simulink model "tetra_mod_qpsk"  (Simulink 8.0)
settings: Solver=FixedStepDiscrete  SolverMode=SingleTasking  StartTime=0.0  StopTime=1.0  RelTol=1e-3
undefined symbols (not defined in the file): figposition, Fs, get, sided, Two
libraries: commsink2 x4, simulink x2, commseqgen2 x2, commcnvcod2 x2, commdigbbndpm3 x2, commfilt2 x2, commrandsrc2 x1, commchan3 x1, dspsnks4 x1, dspvision x1
settings Model: Creator=tisc1101  LastModifiedBy=Dimav
settings DataIOCC: SignalLoggingSaveFormat=ModelDataLogs
settings DebuggingCC: FcnCallInpInsideContextMsg=UseLocalSettings
settings SFSimCC: SimParseCustomCode=off
settings GRTTargetCC: CombineOutputUpdateFcns=off  GRTInterface=on

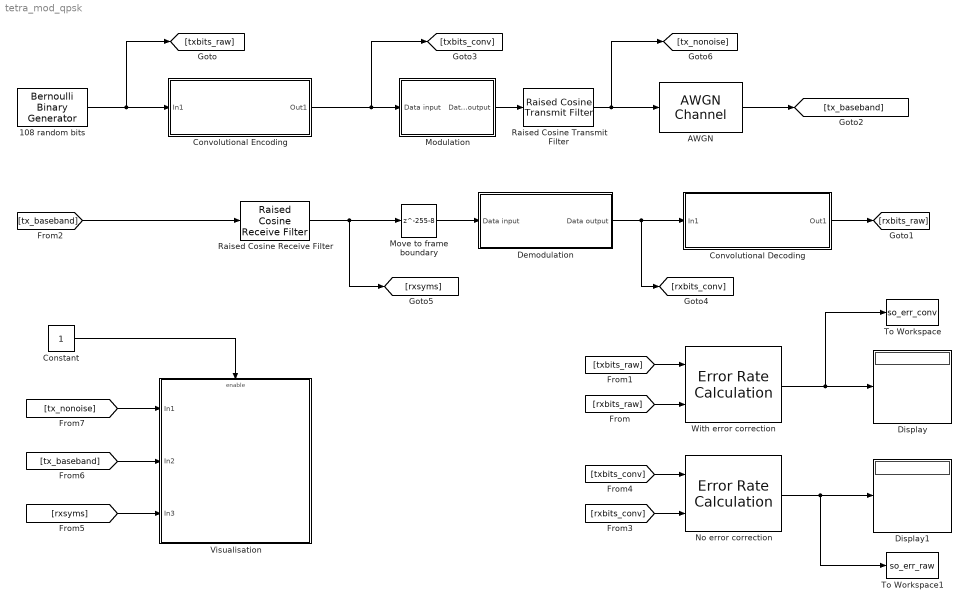
== system tetra_mod_qpsk ==
  108 random bits : commrandsrc2/Bernoulli Binary Generator  P=0.5  seed=61  Ts=1/(36000/512*108)  frameBased=on  sampPerFrame=108  orient=off  outDataType=double
  AWGN : commchan3/AWGN Channel  InputProcessing=Inherited (this choice will be removed - see release notes)  seed=67  noiseMode="Signal to noise ratio  (SNR)"  EbNodB=10  EsNodB=10  SNRdB=-10  bitsPerSym=1  Ps=1  Tsym=1  variance=1
  Constant : Constant
  Convolutional Decoding : Subsystem
  Convolutional Encoding : Subsystem
  Demodulation : Subsystem
  Display : Display
  Display1 : Display
  Modulation : Subsystem
  Move to frame boundary : Delay  DelayLength=255-8  InputProcessing=Inherited
  No error correction : commsink2/Error Rate Calculation  N=216  st_delay=0  cp_mode=Entire frame  subframe=[]  PMode=Port  WsName=ErrorVec  RsMode2=off  stop=off  numErr=100  maxBits=1e6
  Raised Cosine Receive Filter : commfilt2/Raised Cosine Receive Filter  filtType=Square root  N=8  D=4  R=0.35  sampMode=Mute  saveAsFlag=0  rateMode=Downsampling  downFactor=8  downOffset=0  framing=Maintain input frame rate  InputProcessing=Columns as channels (frame based)  checkGain=Normalized  filterGain=2  checkCoeff=off  variableName=rcRxFilt  launchFVT=off  roundingMode=Floor  overflowMode=off
  Raised Cosine Transmit Filter : commfilt2/Raised Cosine Transmit Filter  filtType=Square root  D=4  R=0.35  sampMode=Mute  saveAsFlag=0  N=8  framing=Maintain input frame rate  InputProcessing=Columns as channels (frame based)  checkGain=Normalized  filterGain=1  checkCoeff=off  variableName=rcTxFilt  launchFVT=off  roundingMode=Floor  overflowMode=off
  To Workspace : ToWorkspace  VariableName=so_err_conv  SampleTime=-1  SaveFormat=Structure
  To Workspace1 : ToWorkspace  VariableName=so_err_raw  SampleTime=-1  SaveFormat=Structure
  Visualisation : Subsystem  TreatAsAtomicUnit=on
  With error correction : commsink2/Error Rate Calculation  N=156  st_delay=0  cp_mode=Entire frame  subframe=[]  PMode=Port  WsName=ErrorVec  RsMode2=off  stop=off  numErr=100  maxBits=1e6
  wires:
  Modulation/1(Data output) -> Raised Cosine Transmit Filter/1
  Demodulation/1(Data output) -> [rxbits_conv], Convolutional Decoding/1(In1)
  [rxbits_raw] -> With error correction/2
  With error correction/1 -> Display/1, To Workspace/1
  Raised Cosine Transmit Filter/1 -> AWGN/1, [tx_nonoise]
  [tx_baseband] -> Raised Cosine Receive Filter/1
  Raised Cosine Receive Filter/1 -> Move to frame boundary/1, [rxsyms]
  Move to frame boundary/1 -> Demodulation/1(Data input)
  AWGN/1 -> [tx_baseband]
  Convolutional Encoding/1(Out1) -> Modulation/1(Data input), [txbits_conv]
  Convolutional Decoding/1(Out1) -> [rxbits_raw]
  [txbits_raw] -> With error correction/1
  [rxbits_conv] -> No error correction/2
  No error correction/1 -> Display1/1, To Workspace1/1
  [txbits_conv] -> No error correction/1
  108 random bits/1 -> Convolutional Encoding/1(In1), [txbits_raw]
  Constant/1 -> Visualisation/Enable
  [tx_baseband] -> Visualisation/2(In2)
  [rxsyms] -> Visualisation/3(In3)
  [tx_nonoise] -> Visualisation/1(In1)

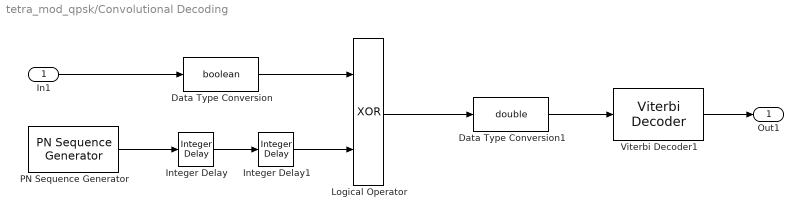
== system tetra_mod_qpsk/Convolutional Decoding ==
  In1 : Inport
  Data Type Conversion : DataTypeConversion  OutDataTypeStr=boolean
  Data Type Conversion1 : DataTypeConversion  OutDataTypeStr=double
  Integer Delay : simulink/Discrete/Integer Delay  NumDelays=215  InputProcessing=Inherited  vinit=0  samptime=-1
  Integer Delay1 : simulink/Discrete/Integer Delay  NumDelays=1  InputProcessing=Inherited  vinit=0  samptime=-1
  Logical Operator : Logic  Operator=XOR  AllPortsSameDT=off  OutDataTypeStr=boolean
  PN Sequence Generator : commseqgen2/PN Sequence Generator  poly=[1 1 1 0 1 1 0 1 1 0 1 1 1 0 0 0 1 0 0 0 0 0 1 1 0 0 1 0 0 0 0 0 1]  ini_sta=[0 1 0 1 0 1 0 1 0 1 0 1 0 1 0 1 0 1 0 1 0 1 0 1 0 1 0 1 0 1 1 1]  outBitMaskSource=Dialog parameter  shift=0  outVarSiz=off  maxOutSizeMode=Dialog parameter  maxOutSize=[10 1]  Ts=1/(36000/512*216)  frameBased=on  sampPerFrame=216  reset=off  bitPackedOutputs=off  outDataType=boolean  numPackedBits=8  bitPackDataSigned=off  bitPackedOutDType=double
  Viterbi Decoder1 : commcnvcod2/Viterbi Decoder  trellis=poly2trellis(7, [171 133])  isPunctured=off  punctureVector=[1; 1; 0; 1; 0; 1]  erasures=off  dectype=Hard decision  runSigValErrCheck=off  nsdecb=3  smWordLength=16  tbdepth=48  opmode=Continuous  reset=off  outDataType=double
  Out1 : Outport
  wires:
  Viterbi Decoder1/1 -> Out1/1
  Logical Operator/1 -> Data Type Conversion1/1
  In1/1 -> Data Type Conversion/1
  PN Sequence Generator/1 -> Integer Delay/1
  Data Type Conversion/1 -> Logical Operator/1
  Data Type Conversion1/1 -> Viterbi Decoder1/1
  Integer Delay/1 -> Integer Delay1/1
  Integer Delay1/1 -> Logical Operator/2

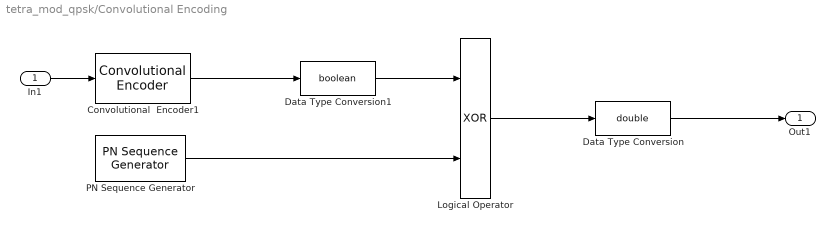
== system tetra_mod_qpsk/Convolutional Encoding ==
  In1 : Inport
  Convolutional  Encoder1 : commcnvcod2/Convolutional Encoder  trellis=poly2trellis(7, [171 133])  opMode=Continuous  DelayedResetAction=off  hasIniStPort=off  hasFinStPort=off  usePuncVector=off  punctureVector=[1; 1; 0; 1; 0; 1]  reset=Unused parameter value
  Data Type Conversion : DataTypeConversion  OutDataTypeStr=double
  Data Type Conversion1 : DataTypeConversion  OutDataTypeStr=boolean
  Logical Operator : Logic  Operator=XOR  AllPortsSameDT=off  OutDataTypeStr=boolean
  PN Sequence Generator : commseqgen2/PN Sequence Generator  poly=[1 1 1 0 1 1 0 1 1 0 1 1 1 0 0 0 1 0 0 0 0 0 1 1 0 0 1 0 0 0 0 0 1]  ini_sta=[0 1 0 1 0 1 0 1 0 1 0 1 0 1 0 1 0 1 0 1 0 1 0 1 0 1 0 1 0 1 1 1]  outBitMaskSource=Dialog parameter  shift=0  outVarSiz=off  maxOutSizeMode=Dialog parameter  maxOutSize=[10 1]  Ts=1/(36000/512*216)  frameBased=on  sampPerFrame=216  reset=off  bitPackedOutputs=off  outDataType=boolean  numPackedBits=8  bitPackDataSigned=off  bitPackedOutDType=double
  Out1 : Outport
  wires:
  In1/1 -> Convolutional  Encoder1/1
  Convolutional  Encoder1/1 -> Data Type Conversion1/1
  PN Sequence Generator/1 -> Logical Operator/2
  Logical Operator/1 -> Data Type Conversion/1
  Data Type Conversion/1 -> Out1/1
  Data Type Conversion1/1 -> Logical Operator/1

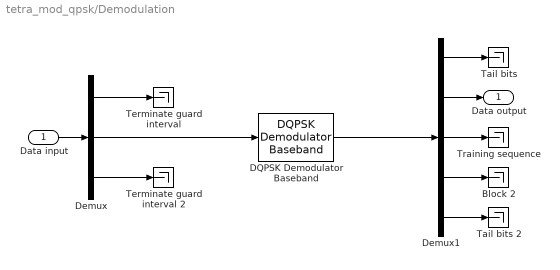
== system tetra_mod_qpsk/Demodulation ==
  Data input : Inport
  Block 2 : Terminator
  DQPSK Demodulator Baseband : commdigbbndpm3/DQPSK Demodulator Baseband  SystemSampleTime=-1  OutType=Bit  Dec=Gray  Ph=pi/4  outDtype1=Inherit via internal rule  outDtype2=Inherit via internal rule
  Demux : Demux  Outputs=[17 231 7]
  Demux1 : Demux  Outputs=[4 216 22 216 4]
  Tail bits : Terminator
  Tail bits 2 : Terminator
  Terminate guard interval : Terminator
  Terminate guard interval 2 : Terminator
  Training sequence : Terminator
  Data output : Outport
  wires:
  Demux/1 -> Terminate guard interval/1
  Demux/3 -> Terminate guard interval 2/1
  Demux/2 -> DQPSK Demodulator Baseband/1
  DQPSK Demodulator Baseband/1 -> Demux1/1
  Demux1/1 -> Tail bits/1
  Demux1/3 -> Training sequence/1
  Demux1/4 -> Block 2/1
  Demux1/5 -> Tail bits 2/1
  Data input/1 -> Demux/1
  Demux1/2 -> Data output/1

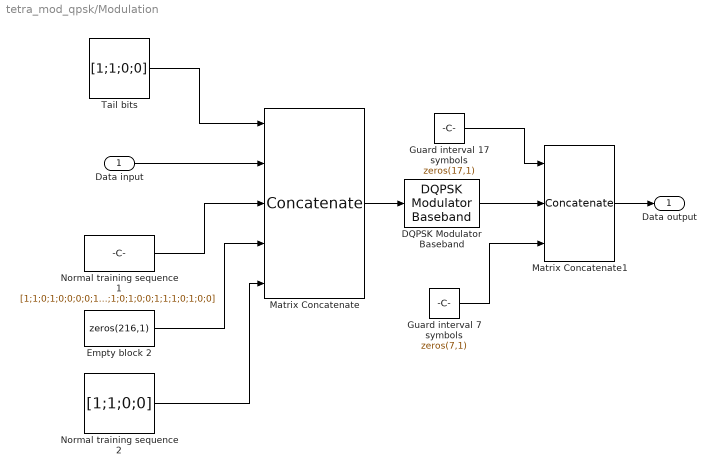
== system tetra_mod_qpsk/Modulation ==
  Data input : Inport
  DQPSK Modulator Baseband : commdigbbndpm3/DQPSK Modulator Baseband  SystemSampleTime=-1  InType=Bit  Enc=Gray  Ph=pi/4  outDtype=double
  Empty block 2 : Constant  Value=zeros(216,1)  VectorParams1D=off
      settings: SamplingMode=Frame based
  Guard interval 17 symbols : Constant  Value=zeros(17,1)  VectorParams1D=off
      settings: SamplingMode=Frame based
  Guard interval 7 symbols : Constant  Value=zeros(7,1)  VectorParams1D=off
      settings: SamplingMode=Frame based
  Matrix Concatenate : Concatenate  NumInputs=5  Mode=Multidimensional array
  Matrix Concatenate1 : Concatenate  NumInputs=3  Mode=Multidimensional array
  Normal training sequence 1 : Constant  Value=[1;1;0;1;0;0;0;0;1;1;1;0;1;0;0;1;1;1;0;1;0;0]  VectorParams1D=off
      settings: SamplingMode=Frame based
  Normal training sequence 2 : Constant  Value=[1;1;0;0]  VectorParams1D=off
      settings: SamplingMode=Frame based
  Tail bits : Constant  Value=[1;1;0;0]  VectorParams1D=off
      settings: SamplingMode=Frame based
  Data output : Outport
  wires:
  Tail bits/1 -> Matrix Concatenate/1
  Data input/1 -> Matrix Concatenate/2
  Normal training sequence 1/1 -> Matrix Concatenate/3
  Empty block 2/1 -> Matrix Concatenate/4
  Normal training sequence 2/1 -> Matrix Concatenate/5
  Matrix Concatenate/1 -> DQPSK Modulator Baseband/1
  Guard interval 17 symbols/1 -> Matrix Concatenate1/1
  DQPSK Modulator Baseband/1 -> Matrix Concatenate1/2
  Guard interval 7 symbols/1 -> Matrix Concatenate1/3
  Matrix Concatenate1/1 -> Data output/1

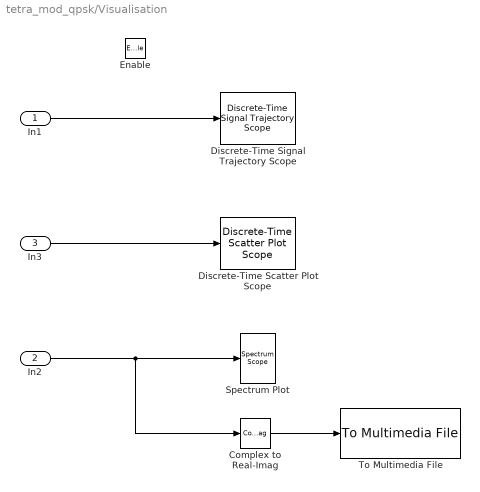
== system tetra_mod_qpsk/Visualisation ==
  In1 : Inport
  In2 : Inport  Port=2
  In3 : Inport  Port=3
  Enable : EnablePort
  Complex to Real-Imag : ComplexToRealImag  Output=Real
  Discrete-Time Scatter Plot Scope : commsink2/Discrete-Time Scatter Plot Scope  Tag=ScatterPlot  sampPerSymb=1  offsetEye=0  numTraces=40  numNewFrames=40  LineMarkers=.  LineColors=b  fading=on  render=on  AxisGrid=on  xMin=-3.3  xMax=3.315  yMin=-3.3  yMax=3.315  inphaseLabel=In-phase Amplitude  quadratureLabel=Quadrature Amplitude  openScopeAtSimStart=on  FrameNumber=off  FigPos=get(0,'defaultfigureposition');  figTitle=Scatter Plot  numLinesMax=8  block_type_=scatter
  Discrete-Time Signal Trajectory Scope : commsink2/Discrete-Time Signal Trajectory Scope  Tag=SignalTrajectory  sampPerSymb=8  offsetEye=0  numTraces=400  numNewFrames=40  LineStyles=-  LineColors=b  fading=on  render=on  AxisGrid=on  xMin=-0.63458380768819  xMax=0.667665055503829  yMin=-0.645070083371635  yMax=0.657178779820385  inphaseLabel=In-phase Amplitude  quadratureLabel=Quadrature Amplitude  openScopeAtSimStart=on  FrameNumber=off  FigPos=get(0,'defaultfigureposition');  figTitle=Signal Trajectory  numLinesMax=8  block_type_=xy
  Spectrum Plot : dspsnks4/Spectrum Scope  ScopeProperties=on  Domain=Frequency  HorizSpan=1  UseBuffer=on  BufferSize=2048  Overlap=0  TreatMby1Signals=M channels  inpFftLenInherit=on  FFTlength=2048  numAvg=5  DisplayProperties=off  AxisGrid=on  Memory=off  FrameNumber=on  AxisLegend=off  AxisZoom=off  OpenScopeAtSimStart=on  OpenScopeImmediately=off  FigPos="figposition([33  30 30 25])"  AxisProperties=off  XUnits=Hertz  XRange=Two-sided ((-Fs/2...Fs/2])  XDisplay=0  InheritXIncr=on  XIncr=1.0  XLabel=Samples  XLimit=Auto  YUnits=dBW/Hertz  XMax=1  XMin=0  YLabel=Magnitude, dB  LineProperties=off  LineStyles=--  wintypeSpecScope=Hann  RsSpecScope=50  betaSpecScope=5  winsampSpecScope=Periodic  XAxisParamsVer=6.9  isFrameUpgraded=on
      settings: YMin=-100  YMax=30
  To Multimedia File : dspvision/To Multimedia File  outputFilename=output.wav  streamSelection=Audio only  videoCompressor=None (uncompressed)  audioCompressor=None (uncompressed)  imagePorts=Separate color signals  fileType=WAV  audioDatatype=32-bit float  fourcc=RGB
  wires:
  Complex to Real-Imag/1 -> To Multimedia File/1
  In2/1 -> Complex to Real-Imag/1, Spectrum Plot/1
  In1/1 -> Discrete-Time Signal Trajectory Scope/1
  In3/1 -> Discrete-Time Scatter Plot Scope/1
